simulink model "simulink_model_to_build_s_function"  (R2019b)
settings: Solver=VariableStepAuto  StartTime=0.0  StopTime=inf  RelTol=1e-3
libraries: dspsrcs4 x2, sldrtlib x1
settings Model: Creator=mandl  LastModifiedBy=mandl

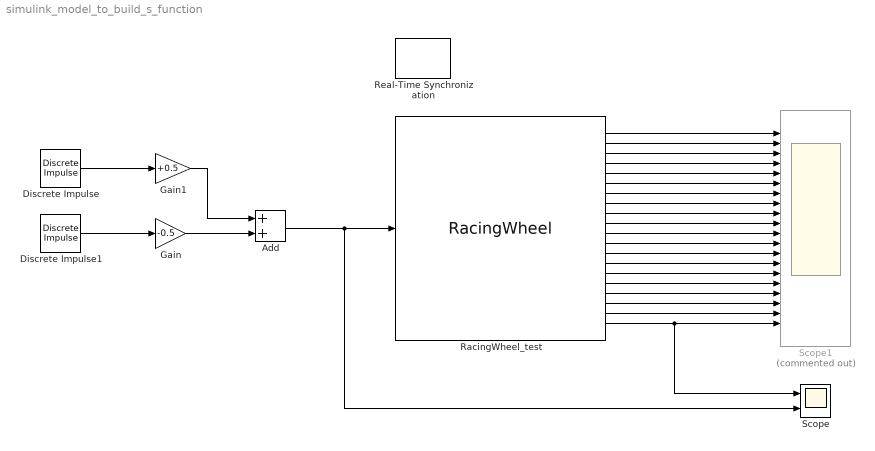
== system simulink_model_to_build_s_function ==
  Add : Sum
  Discrete Impulse : dspsrcs4/Discrete  Impulse  Delay=500  SampleTime=0.01  FrameSample=1  OutputFrames=off  dataType=double  isSigned=on  wordLen=16  udDataType=sfix(16)  fracBitsMode=Best precision  numFracBits=15  OutDataTypeStr=double  LastOutDataTypeStr=double
  Discrete Impulse1 : dspsrcs4/Discrete  Impulse  Delay=1000  SampleTime=0.01  FrameSample=1  OutputFrames=off  dataType=double  isSigned=on  wordLen=16  udDataType=sfix(16)  fracBitsMode=Best precision  numFracBits=15  OutDataTypeStr=double  LastOutDataTypeStr=double
  Gain : Gain  Gain=-0.5
  Gain1 : Gain  Gain=+0.5
  RacingWheel_test : S-Function  InitFcn=try, set_param(gcb,'FunctionName','RacingWheel'), end  FunctionName=RacingWheel  Parameters=0.01  SFunctionModules=RacingWheel_wrapper  SFunctionDeploymentMode=off  EnableBusSupport=off  mask(S-Function Builder){}
      mask help: Simulink:masks:SFunctionBuilder_MD
      mask init:
      | val = [[.9  0.75 0.75 1 1 .9 .9 1]',[1 1 0.75 0.75 .9 .9 1 .9]'];try , sys = get_param(gcb,'SfunBuilderFcnName');if isempty(sys), sys = get_param(gcb,'FunctionName'); end,catch, sys = get_param(gcb,'FunctionName'); end
      settings: CopyFcn=set_param(gcbh,'LinkStatus','none')  PreSaveFcn=try, set_param(gcb,'FunctionName','RacingWheel'), end  OpenFcn=sfunctionwizard(gcbh)
      mask Display: plot(val(:,1),val(:,2)),disp(sys), port_label('input',1,'FF_bias'), port_label('output',1,'gearup'), port_label('output',2,'geardown'), port_label('output',3,'ST'), port_label('output',4,'SE'), port_label('output',5,'X'), port_label('output',6,'O'), port_label('output',7,'Square'), port_label('output',8,'Triangle'), port_label('output',9,'L2'), port_label('output',10,'R2'), port_label('output',11,'L3'), port_label('output',12,'R3'), port_label('output',13,'DPadDown'), port_label('output',14,'DPadUp'), port_label('output',15,'DPadLeft'), port_label('output',16,'DPadRight'), port_label('output',17,'throttle'), port_label('output',18,'brake'), port_label('output',19,'clutch'), port_label('output',20,'angle')
  Real-Time Synchronization : sldrtlib/Real-Time Synchronization  SampleTime=0.01  MaxMissedTicks=inf  ShowMissedTicks=off  YieldWhenWaiting=on
  Scope : Scope  NumInputPorts=2
  Scope1 : Scope  Commented=on  NumInputPorts=20
  wires:
  RacingWheel_test/1 -> Scope1/1
  RacingWheel_test/2 -> Scope1/2
  RacingWheel_test/3 -> Scope1/3
  RacingWheel_test/4 -> Scope1/4
  RacingWheel_test/5 -> Scope1/5
  RacingWheel_test/6 -> Scope1/6
  RacingWheel_test/7 -> Scope1/7
  RacingWheel_test/8 -> Scope1/8
  RacingWheel_test/9 -> Scope1/9
  RacingWheel_test/10 -> Scope1/10
  RacingWheel_test/11 -> Scope1/11
  RacingWheel_test/12 -> Scope1/12
  RacingWheel_test/13 -> Scope1/13
  RacingWheel_test/14 -> Scope1/14
  RacingWheel_test/15 -> Scope1/15
  RacingWheel_test/16 -> Scope1/16
  RacingWheel_test/17 -> Scope1/17
  RacingWheel_test/18 -> Scope1/18
  RacingWheel_test/19 -> Scope1/19
  RacingWheel_test/20 -> Scope/1, Scope1/20
  Discrete Impulse/1 -> Gain1/1
  Discrete Impulse1/1 -> Gain/1
  Gain/1 -> Add/2
  Gain1/1 -> Add/1
  Add/1 -> Scope/2, RacingWheel_test/1
